simulink model "offline_csws_model"  (R2021a)
settings: Solver=FixedStepDiscrete  StartTime=0.0  StopTime=62  FixedStep=1  RelTol=1e-3
model workspace (MAT data in the model file):
  t = 0
libraries: CSWLibrary x2
settings Model: Creator=Martin  LastModifiedBy=Martin
settings SolverCC: ConcurrentTasks=on  PositivePriorityOrder=on
settings OptimizationCC: BlockReduction=off  OptimizeBlockIOStorage=off
settings DebuggingCC: TasksWithSamePriorityMsg=none
settings HardwareCC: ProdBitPerLong=64  ProdLongLongMode=on  ProdHWDeviceType=Intel->x86-64 (Linux 64)
settings RTWCC: Description=Simulink Real-Time  SystemTargetFile=slrealtime.tlc  TemplateMakefile=slrealtime_default_tmf  Toolchain=Simulink Real-Time Toolchain  BuildConfiguration=Faster Runs  CodeExecutionProfiling=on  TargetLang=C++

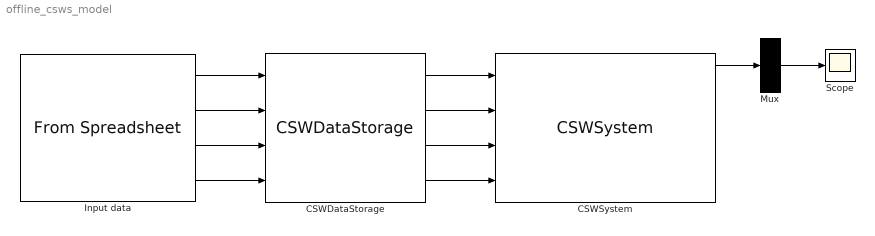
== system offline_csws_model ==
  CSWDataStorage : CSWLibrary/CSWDataStorage
      settings: SourceProductName=Curve Speed Warning System Toolbox
  CSWSystem : CSWLibrary/CSWSystem  predictionTime=5  maximumLateralAcceleration=5.9  safeLimit=60  warningValue=1  lowerRadius=20  upperRadius=600  visualizeTrajectory=on  saveResults=on  simulationResultsFile=results.xlsx
      settings: SourceProductName=Curve Speed Warning System Toolbox
  Input data : FromSpreadsheet  FileName=<PATH-TO-FILE>\exampleData.xlsx  SheetName=Sheet  Range=A1:D64  TreatFirstColumnAs=Data  SampleTime=-1  OutputAfterLastPoint=Ground value
  Mux : Mux  Inputs=1
  Scope : Scope
  wires:
  Input data/3 -> CSWDataStorage/3
  Input data/1 -> CSWDataStorage/1
  Input data/2 -> CSWDataStorage/2
  Input data/4 -> CSWDataStorage/4
  CSWDataStorage/4 -> CSWSystem/4
  CSWDataStorage/3 -> CSWSystem/3
  CSWDataStorage/2 -> CSWSystem/2
  CSWDataStorage/1 -> CSWSystem/1
  CSWSystem/1 -> Mux/1
  Mux/1 -> Scope/1
